simulink model "Simul_LQR"  (R2020b)
settings: Solver=VariableStepAuto  StartTime=0.0  StopTime=50  RelTol=1e-3
values from neighbouring files (symbols this model uses):
  h = 0.05    [Unity3Dsimulacion.m]
  X0 = [0 0 0 0]    [Unity3Dsimulacion.m]
libraries: cstblocks x1
settings Model: PauseTimes=0  Creator=Eduard  LastModifiedBy=Eduard

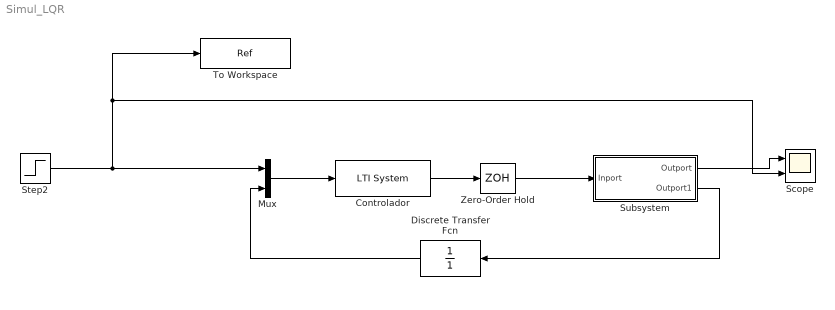
== system Simul_LQR ==
  Controlador : cstblocks/LTI System  sys=MLc  IC=[]
  Discrete Transfer Fcn : DiscreteTransferFcn  Denominator=[1]  SampleTime=h
  Mux : Mux  Inputs=2
  Scope : Scope  NumInputPorts=2
  Step2 : Step  Time=0  After=0.5  SampleTime=0
  Subsystem : Subsystem
  To Workspace : ToWorkspace  VariableName=Ref  SaveFormat=Structure With Time  SampleTime=-1
  Zero-Order Hold : ZeroOrderHold  SampleTime=h
  wires:
  Controlador/1 -> Zero-Order Hold/1
  Mux/1 -> Controlador/1
  Step2/1 -> Mux/1, To Workspace/1, Scope/2
  Subsystem/1(Outport) -> Scope/1
  Zero-Order Hold/1 -> Subsystem/1(Inport)
  Subsystem/2(Outport1) -> Discrete Transfer Fcn/1
  Discrete Transfer Fcn/1 -> Mux/2

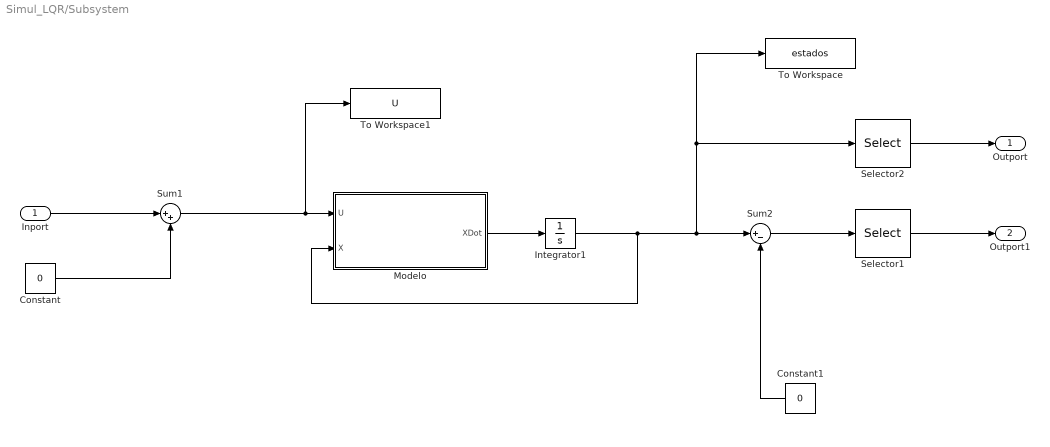
== system Simul_LQR/Subsystem ==
  Inport : Inport
  Constant : Constant  Value=0
  Constant1 : Constant  Value=0
  Integrator1 : Integrator  InitialCondition=X0
  Modelo : MATLAB Function  TreatAsAtomicUnit=on
  Selector1 : Selector  InputPortWidth=4  IndexOptions=Index vector (dialog)  Indices=[2]  OutputSizes=1
  Selector2 : Selector  InputPortWidth=4  IndexOptions=Index vector (dialog)  Indices=[2]  OutputSizes=1
  Sum1 : Sum  Inputs=|++
  Sum2 : Sum  Inputs=|+-
  To Workspace : ToWorkspace  VariableName=estados  SaveFormat=Structure With Time  SampleTime=-1
  To Workspace1 : ToWorkspace  VariableName=U  SaveFormat=Structure With Time  SampleTime=h
  Outport : Outport
  Outport1 : Outport  Port=2
  wires:
  Constant/1 -> Sum1/2
  Inport/1 -> Sum1/1
  Constant1/1 -> Sum2/2
  Sum2/1 -> Selector1/1
  Selector2/1 -> Outport/1
  Selector1/1 -> Outport1/1
  Modelo/1(XDot) -> Integrator1/1
  Integrator1/1 -> Modelo/2(X), To Workspace/1, Selector2/1, Sum2/1
  Sum1/1 -> To Workspace1/1, Modelo/1(U)

== matlab function Simul_LQR/Subsystem/Modelo ==
  data: XDot output; U input; X input
function XDot = ball_and_beam_model(U,X)
%#codegen
% Constants of the model
[m,J,r,g]           = deal(0.1,0.025,0.01,9.807);

%% State space model
% x1 = theta, x2  = x, x3 = thetadot, x4 = xdot
[X1,X2,X3,X4]= deal(X(1),X(2),X(3),X(4));

% Inertia matrix
D           = [m*r^2+m*X2^2+J, -m*r; -m*r, m];

% Coriolis and centrifugal forces
H           = [2*m*X2*X4*X3; -m*X2*X3^2];

% Gravity forces
G           = [m*g*X2*cos(X1)-m*g*r*sin(X1); m*g*sin(X1)];

% Generalized effort
E           = [U; 0];

% Derivatives of states
XDot        = [X3; X4; D\(E-H-G)];
end
